simulink model "ADCS_sim"  (R2018b)
settings: Solver=VariableStepAuto  StartTime=0.0  StopTime=T
values from neighbouring files (symbols this model uses):
  A_i = [A_sc(1); A_sc(2); A_sc(3); A_sc(1); A_sc(2); A_sc(3);            A_sa; A_sa; A_sa; A_sa]'    [data_setup.m]
  G = [1 10 1e-4 1e-4 1e-4 1e-4]    [main.m]
  mag_res = [1; 1; 1]*1e-3    [data_setup.m]
  n = length(t)    [main.m]
  n_i = [eye(3), -eye(3), n_sa, -n_sa, n_sa, -n_sa]    [data_setup.m]
  P = zeros(18,18,nF)    [main_test_ekf.m]
  r_i = [CG_1, CG_2, CG_3, CG_4, CG_5, CG_6, CG_7, CG_8, CG_9, CG_10]    [data_setup.m]
  rhoD = ones(1,10)*0.1    [data_setup.m]
  rhoS = [ones(1,6)*0.5, ones(1,4)*0.8]    [data_setup.m]
undefined symbols (not defined in the file or in its folder): A, a, alp_w, Ar, Ar_star, B, C, e, epsilon, fov_star, fov_sun, g1_0, H0, in, Ir, Ixyz, L, mi, n_star_sens, n_sun, n_sun_sens, omega0, omegaE, R_e, R_sun, RAAN, rate_mag, rate_star, rate_sun, sig_mag, sig_star, sig_sun, star_cat, th0
libraries: simulink_extras x9, vrlib x6, dspmathops x5, simulink x5, sharedutil x2, dspmtrx3 x1, dspfactors x1
(part 2 of 2)

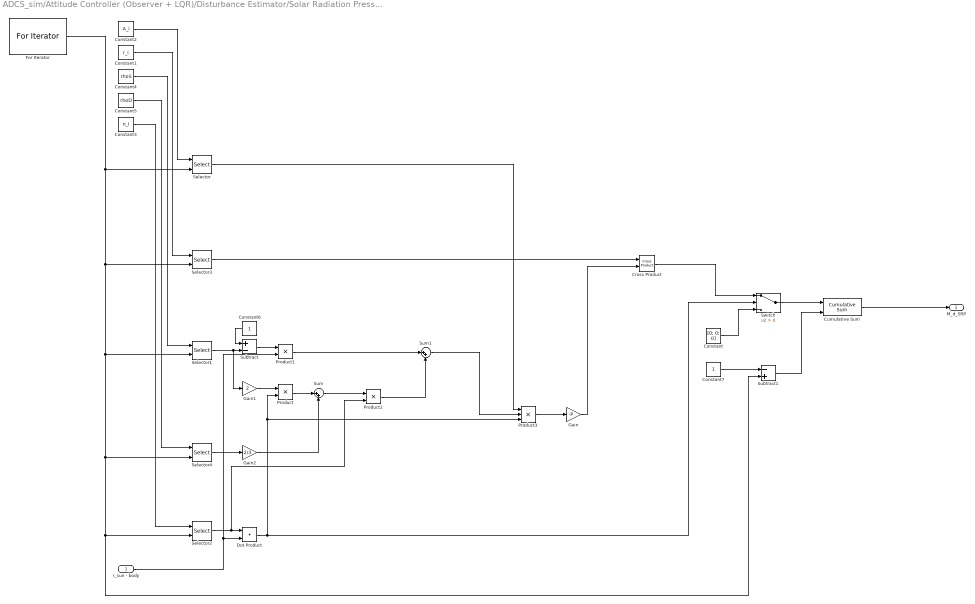
== system ADCS_sim/Attitude Controller (Observer + LQR)/Disturbance Estimator/Solar Radiation Pressure ==
  r_sun - body : Inport
  Constant : Constant  Value=[0; 0; 0]
  Constant1 : Constant  Value=r_i
  Constant2 : Constant  Value=A_i
  Constant3 : Constant  Value=n_i
  Constant4 : Constant  Value=rhoS
  Constant5 : Constant  Value=rhoD
  Constant6 : Constant
  Constant7 : Constant
  Cross Product : vrlib/Utilities/Cross Product
      settings: SourceProductBaseCode=VR
  Cumulative Sum : dspmathops/Cumulative Sum  dim=Channels (running sum)  reset_popup=Falling edge  roundingMode=Floor  overflowMode=off  outputDataTypeStr=Inherit: Same as accumulator  outputMin=[]  outputMax=[]  outputLastDataTypeStr=Inherit: Same as accumulator
      settings: SourceProductName=DSP System Toolbox
  Dot Product : DotProduct  InputSameDT=on  OutDataTypeStr=Inherit: Inherit via internal rule
  For Iterator : ForIterator  IterationLimit=length(A_i)
  Gain : Gain  Gain=-P
  Gain1 : Gain  Gain=2
  Gain2 : Gain  Gain=2/3
  Product : Product
  Product1 : Product
  Product2 : Product
  Product3 : Product  Inputs=3
  Selector{,1..4} (5 alike) : Selector  NumberOfDimensions=2  InputPortWidth=3  IndexOptions=Select all,Index vector (port)  Indices=[1 3],1  OutputSizes=1,1
  Subtract : Sum  Inputs=+-
  Subtract1 : Sum  Inputs=-+
  Sum : Sum  Inputs=|++
  Sum1 : Sum  Inputs=|++
  Switch : Switch  Criteria=u2 > Threshold
  M_d_SRP : Outport
  wires:
  For Iterator/1 -> Selector/2, Selector3/2, Subtract1/2, Selector2/2, Selector4/2, Selector1/2
  Selector/1 -> Product3/1
  Selector3/1 -> Cross Product/1
  Constant3/1 -> Selector2/1
  Selector2/1 -> Product2/2, Dot Product/1
  Constant1/1 -> Selector3/1
  Constant2/1 -> Selector/1
  r_sun - body/1 -> Product1/2, Dot Product/2
  Constant4/1 -> Selector1/1
  Constant5/1 -> Selector4/1
  Selector1/1 -> Subtract/2, Gain1/1
  Constant6/1 -> Subtract/1
  Subtract/1 -> Product1/1
  Dot Product/1 -> Product/2, Product3/3, Switch/2
  Gain1/1 -> Product/1
  Selector4/1 -> Gain2/1
  Product/1 -> Sum/1
  Gain2/1 -> Sum/2
  Sum/1 -> Product2/1
  Product1/1 -> Sum1/1
  Product2/1 -> Sum1/2
  Sum1/1 -> Product3/2
  Product3/1 -> Gain/1
  Gain/1 -> Cross Product/2
  Constant/1 -> Switch/3
  Cross Product/1 -> Switch/1
  Switch/1 -> Cumulative Sum/1
  Subtract1/1 -> Cumulative Sum/2
  Constant7/1 -> Subtract1/1
  Cumulative Sum/1 -> M_d_SRP/1

== system ADCS_sim/Attitude Controller (Observer + LQR)/Disturbance Estimator/Subsystem3 ==
  A_bn : Inport
  B - inert FOR : Inport  Port=2
  Constant6 : Constant  Value=mag_res
  Cross Product : vrlib/Utilities/Cross Product
      settings: SourceProductBaseCode=VR
  Matrix Multiply1 : Product  Multiplication=Matrix(*)
  M_mag : Outport
  wires:
  Matrix Multiply1/1 -> Cross Product/2  "b - body FOR"
  B - inert FOR/1 -> Matrix Multiply1/2
  Constant6/1 -> Cross Product/1
  Cross Product/1 -> M_mag/1
  A_bn/1 -> Matrix Multiply1/1

== system ADCS_sim/Attitude Controller (Observer + LQR)/Observer and Controller /omega estimator ==
  state : Inport
  Constant : Constant
  Constant1 : Constant  Value=n
  Demux : Demux  Outputs=6
  Gain : Gain  Gain=-1
  Gain1 : Gain  Gain=-1
  Gain2 : Gain  Gain=-1
  Matrix Multiply : Product  Multiplication=Matrix(*)
  Mux{,1..3} (4 alike) : Mux  Inputs=3
  Sum : Sum  Inputs=|++
  Vector Concatenate : Concatenate  NumInputs=3  Mode=Multidimensional array  ConcatenateDimension=2
  omega : Outport
  wires:
  state/1 -> Demux/1
  Constant/1 -> Mux/1, Mux1/2, Mux2/3
  Gain/1 -> Mux/2
  Demux/3 -> Mux1/1, Gain/1
  Demux/2 -> Gain2/1, Mux/3
  Gain1/1 -> Mux1/3
  Demux/1 -> Mux2/2, Gain1/1
  Gain2/1 -> Mux2/1
  Mux1/1 -> Vector Concatenate/2
  Mux/1 -> Vector Concatenate/1
  Mux2/1 -> Vector Concatenate/3
  Vector Concatenate/1 -> Matrix Multiply/1
  Sum/1 -> Mux3/3
  Demux/4 -> Mux3/1
  Demux/5 -> Mux3/2
  Demux/6 -> Sum/1
  Constant1/1 -> Sum/2
  Mux3/1 -> Matrix Multiply/2
  Matrix Multiply/1 -> omega/1

== system ADCS_sim/Orbital Mechanics/Orbital Mechanics evolut./Radius ==
  theta : Inport
  a : Inport  Port=2
  e : Inport  Port=3
  Constant2 : Constant
  Cos : Trigonometry  Operator=cos
  Divide : Product  Inputs=*/
  Multiply : Product
  Product : Product
  Square : Math  Operator=square  SaturateOnIntegerOverflow=on
  Subtract : Sum  Inputs=+-
  Sum : Sum  Inputs=|++
  R : Outport
  wires:
  Multiply/1 -> Divide/1
  Product/1 -> Sum/2
  Constant2/1 -> Sum/1, Subtract/1
  e/1 -> Product/1, Square/1
  a/1 -> Multiply/1
  Square/1 -> Subtract/2
  theta/1 -> Cos/1
  Divide/1 -> R/1
  Subtract/1 -> Multiply/2
  Sum/1 -> Divide/2
  Cos/1 -> Product/2

== system ADCS_sim/Orbital Mechanics/Orbital Mechanics evolut./True An. evolut. ==
  a : Inport
  e : Inport  Port=2
  mi : Inport  Port=3
  " theta " : Inport  Port=4
  Constant4 : Constant  Value=3
  Constant5 : Constant
  Constant6 : Constant  Value=3/2
  Cos : Trigonometry  Operator=cos
  Divide : Product  Inputs=*/
  Divide1 : Product  Inputs=*/
  Power : Math  Operator=pow  SaturateOnIntegerOverflow=on
  Power1 : Math  Operator=pow  SaturateOnIntegerOverflow=on
  Product : Product
  Product1 : Product
  Sqrt : Sqrt  SaturateOnIntegerOverflow=on
  Square : Math  Operator=square  SaturateOnIntegerOverflow=on
  Square1 : Math  Operator=square  SaturateOnIntegerOverflow=on
  Subtract : Sum  Inputs=+-
  Sum : Sum  Inputs=|++
  theta_dot : Outport
  wires:
  Constant5/1 -> Subtract/1, Sum/2
  Square1/1 -> Subtract/2  "e^2"
  Constant4/1 -> Power/2
  Product/1 -> Sum/1  "e*cos(th)"
  e/1 -> Square1/1, Product/1
  Divide/1 -> Sqrt/1
  " theta "/1 -> Cos/1
  Power/1 -> Divide/2
  Sum/1 -> Square/1
  Sqrt/1 -> Product1/1  "n"
  Product1/1 -> Divide1/1  "Num"
  Power1/1 -> Divide1/2  "Den"
  Divide1/1 -> theta_dot/1
  Constant6/1 -> Power1/2
  a/1 -> Power/1
  Subtract/1 -> Power1/1
  Cos/1 -> Product/2
  Square/1 -> Product1/2
  mi/1 -> Divide/1
